simulink model "Problem6final"  (R2023b)
settings: Solver=VariableStepAuto  StartTime=0.0  StopTime=20  RelTol=1e-3
values from neighbouring files (symbols this model uses):
  G_den6 = [1 2 3 4 1]    [d_56.m]
  G_num6 = [4 3 2 1]    [d_56.m]
settings Model: Creator=Poopy  LastModifiedBy=Poopy

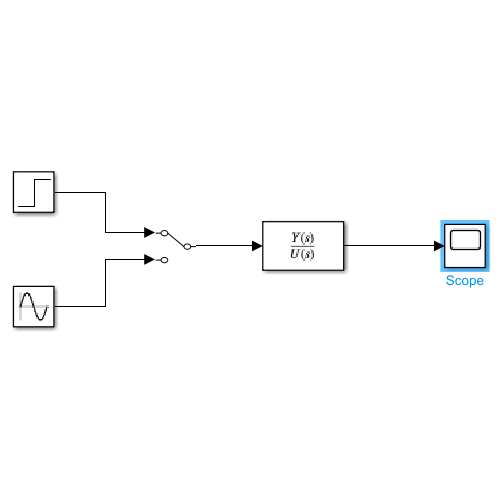
[thumbnail: Simulink's stored preview of the top-level diagram]
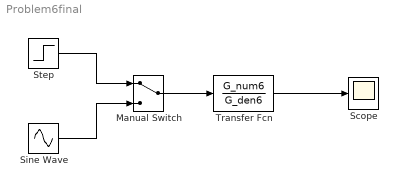
== system Problem6final ==
  Manual Switch : ManualSwitch
  Scope : Scope
  Sine Wave : Sin  SampleTime=0
  Step : Step  Time=0  SampleTime=0
  Transfer Fcn : TransferFcn  Numerator=G_num6  Denominator=G_den6
  wires:
  Sine Wave/1 -> Manual Switch/2
  Transfer Fcn/1 -> Scope/1
  Manual Switch/1 -> Transfer Fcn/1
  Step/1 -> Manual Switch/1
